simulink model "largeanal"  (R2018b)
settings: Solver=VariableStepAuto  StartTime=0.0  StopTime=10.0  RelTol=1e-3
settings Model: Creator=Ramiro  LastModifiedBy=Ramiro

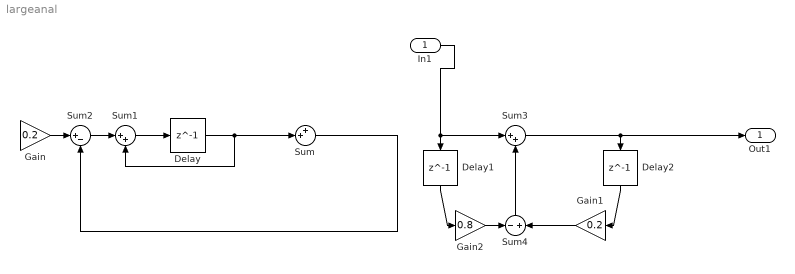
== system largeanal ==
  In1 : Inport
  Delay : Delay  DelayLength=1  InitialCondition=0
  Delay1 : Delay  DelayLength=1  InitialCondition=0
  Delay2 : Delay  DelayLength=1  InitialCondition=0
  Gain : Gain  Gain=0.2
  Gain1 : Gain  Gain=0.2
  Gain2 : Gain  Gain=0.8
  Sum : Sum  Inputs=++|
  Sum1 : Sum  Inputs=|++
  Sum2 : Sum  Inputs=|+-
  Sum3 : Sum  Inputs=|++
  Sum4 : Sum  Inputs=-+
  Out1 : Outport
  wires:
  Delay/1 -> Sum1/2, Sum/2
  Sum/1 -> Sum2/2
  Sum1/1 -> Delay/1
  ? -> Sum/1, Gain/1
  Gain/1 -> Sum2/1
  Sum2/1 -> Sum1/1
  Sum3/1 -> Out1/1, Delay2/1
  Sum4/1 -> Sum3/2
  Delay2/1 -> Gain1/1
  Gain1/1 -> Sum4/2
  Delay1/1 -> Gain2/1
  Gain2/1 -> Sum4/1
  In1/1 -> Sum3/1, Delay1/1
